simulink model "Evaporator"  (R2022b)
settings: Solver=ode45  StartTime=0.0  StopTime=30  RelTol=1e-3
undefined symbols (not defined in the file): h3, tc, tcw12
settings Model: Creator=YJT  LastModifiedBy=YJT

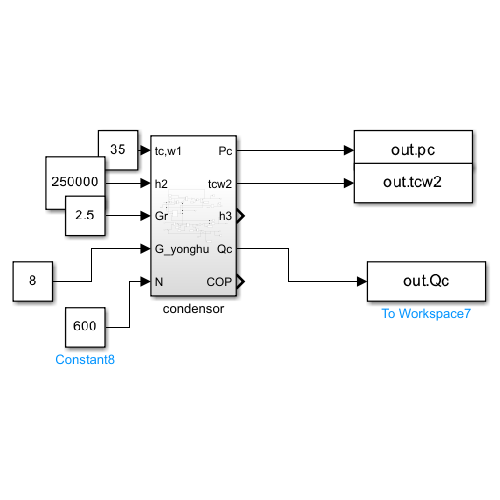
[thumbnail: Simulink's stored preview of the top-level diagram]
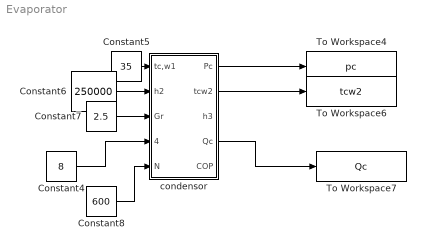
== system Evaporator ==
  Constant4 : Constant  Value=8
  Constant5 : Constant  Value=35
  Constant6 : Constant  Value=250000
  Constant7 : Constant  Value=2.5
  Constant8 : Constant  Value=600
  To Workspace4 : ToWorkspace  VariableName=pc  SaveFormat=Timeseries  SampleTime=-1
  To Workspace6 : ToWorkspace  VariableName=tcw2  SaveFormat=Timeseries  SampleTime=-1
  To Workspace7 : ToWorkspace  VariableName=Qc  SaveFormat=Timeseries  SampleTime=-1
  condensor : Subsystem
  wires:
  Constant4/1 -> condensor/4(G_yonghu)
  Constant5/1 -> condensor/1(tc,w1)
  Constant6/1 -> condensor/2(h2)
  Constant7/1 -> condensor/3(Gr)
  Constant8/1 -> condensor/5(N)
  condensor/1(Pc) -> To Workspace4/1
  condensor/4(Qc) -> To Workspace7/1
  condensor/2(tcw2) -> To Workspace6/1

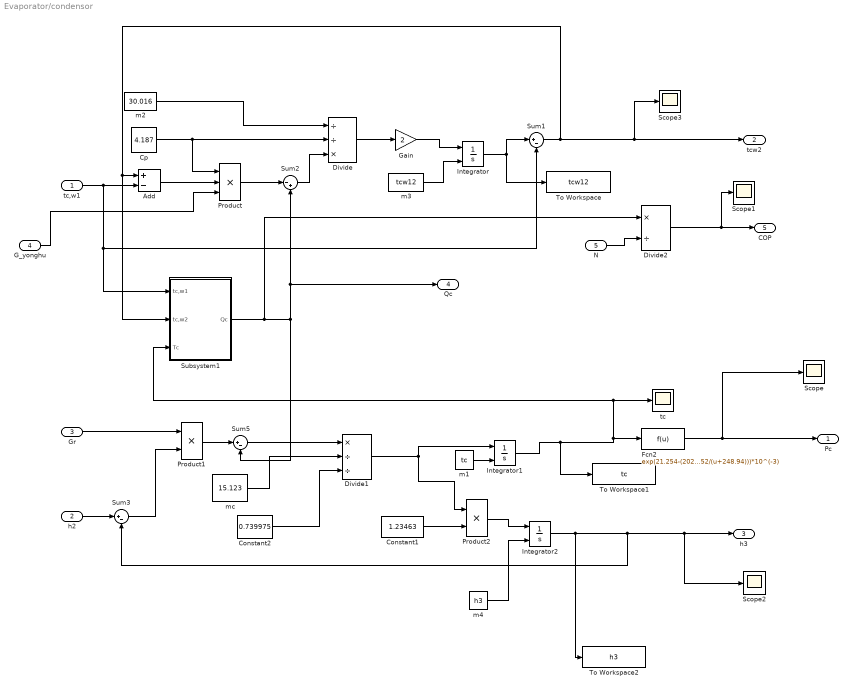
== system Evaporator/condensor ==
  tc,w1 : Inport
  h2 : Inport  Port=2
  Gr : Inport  Port=3
  G_yonghu : Inport  Port=4
  N : Inport  Port=5
  Add : Sum  Inputs=+-
  Constant1 : Constant  Value=1.23463
  Constant2 : Constant  Value=0.739975
  Cp : Constant  Value=4.187
  Divide : Product  Inputs=//*
  Divide1 : Product  Inputs=*//
  Divide2 : Product  Inputs=*/
  Fcn2 : Fcn  Expr=exp(21.254-(2025.452/(u+248.94)))*10^(-3)
  Gain : Gain  Gain=2
  Integrator : Integrator  InitialConditionSource=external
  Integrator1 : Integrator  InitialConditionSource=external
  Integrator2 : Integrator  InitialConditionSource=external
  Product : Product  Inputs=3
  Product1 : Product
  Product2 : Product
  Scope{,1..3} (4 alike) : Scope
  Subsystem1 : Subsystem
  Sum1 : Sum  Inputs=|+-
  Sum2 : Sum  Inputs=|-+
  Sum3 : Sum  Inputs=|+-
  Sum5 : Sum  Inputs=|+-
  To Workspace : ToWorkspace  VariableName=tcw12  SaveFormat=Timeseries  SampleTime=-1
  To Workspace1 : ToWorkspace  VariableName=tc  SaveFormat=Timeseries  SampleTime=-1
  To Workspace2 : ToWorkspace  VariableName=h3  SaveFormat=Timeseries  SampleTime=-1
  m1 : Constant  Value=tc
  m2 : Constant  Value=30.016
  m3 : Constant  Value=tcw12
  m4 : Constant  Value=h3
  mc : Constant  Value=15.123
  tc : Scope
  Pc : Outport
  tcw2 : Outport  Port=2
  h3 : Outport  Port=3
  Qc : Outport  Port=4
  COP : Outport  Port=5
  wires:
  Product1/1 -> Sum5/1
  Sum3/1 -> Product1/2
  Sum1/1 -> Scope3/1, tcw2/1, Subsystem1/2(tc,w2), Add/1
  Gr/1 -> Product1/1
  Integrator2/1 -> To Workspace2/1, Scope2/1, h3/1, Sum3/2
  Constant2/1 -> Divide1/3
  Gain/1 -> Integrator/1
  tc,w1/1 -> Add/2, Subsystem1/1(tc,w1), Sum1/2
  Fcn2/1 -> Scope/1, Pc/1
  Product2/1 -> Integrator2/1
  Integrator/1 -> Sum1/1, To Workspace/1
  m2/1 -> Divide/1
  Cp/1 -> Product/1, Divide/2
  Constant1/1 -> Product2/2
  G_yonghu/1 -> Product/3
  Divide1/1 -> Integrator1/1, Product2/1
  Divide/1 -> Gain/1
  h2/1 -> Sum3/1
  Product/1 -> Sum2/1
  Add/1 -> Product/2
  Sum5/1 -> Divide1/1
  Sum2/1 -> Divide/3
  mc/1 -> Divide1/2
  m1/1 -> Integrator1/2
  Integrator1/1 -> To Workspace1/1, tc/1, Subsystem1/3(Tc), Fcn2/1
  m3/1 -> Integrator/2
  m4/1 -> Integrator2/2
  Divide2/1 -> Scope1/1, COP/1
  Subsystem1/1(Qc) -> Divide2/1, Sum5/2, Qc/1, Sum2/2
  N/1 -> Divide2/2

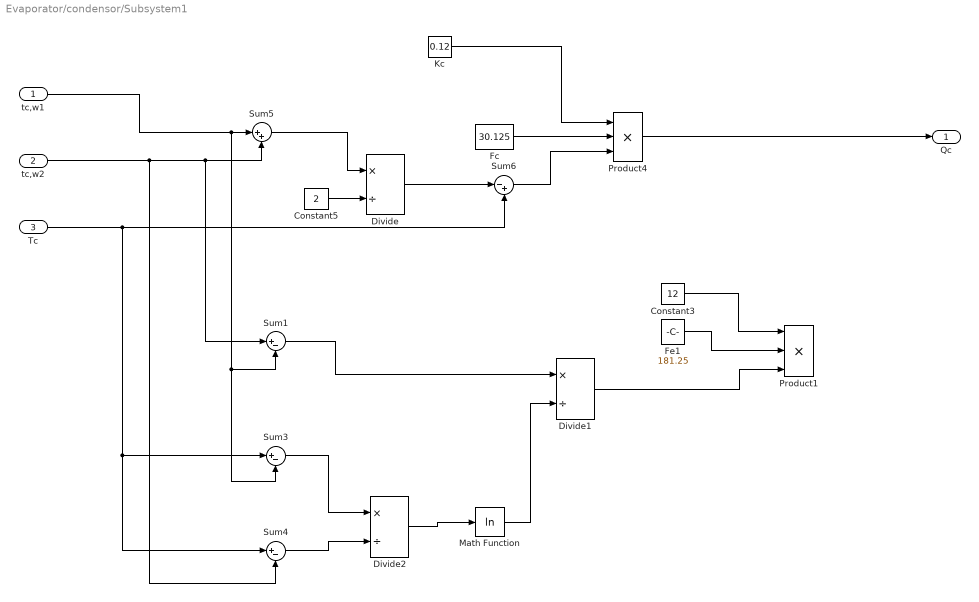
== system Evaporator/condensor/Subsystem1 ==
  tc,w1 : Inport
  tc,w2 : Inport  Port=2
  Tc : Inport  Port=3
  Constant3 : Constant  Value=12
  Constant5 : Constant  Value=2
  Divide : Product  Inputs=*/
  Divide1 : Product  Inputs=*/
  Divide2 : Product  Inputs=*/
  Fc : Constant  Value=30.125
  Fe1 : Constant  Value=181.25
  Kc : Constant  Value=0.12
  Math Function : Math  Operator=log
  Product1 : Product  Inputs=3
  Product4 : Product  Inputs=3
  Sum1 : Sum  Inputs=|+-
  Sum3 : Sum  Inputs=|+-
  Sum4 : Sum  Inputs=|+-
  Sum5 : Sum  Inputs=|++
  Sum6 : Sum  Inputs=|-+
  Qc : Outport
  wires:
  Divide/1 -> Sum6/1
  Fc/1 -> Product4/2
  Sum6/1 -> Product4/3
  Tc/1 -> Sum4/1, Sum3/1, Sum6/2
  Constant5/1 -> Divide/2
  Kc/1 -> Product4/1
  Sum5/1 -> Divide/1
  Sum3/1 -> Divide2/1
  Divide2/1 -> Math Function/1
  tc,w1/1 -> Sum3/2, Sum1/2, Sum5/1
  Sum1/1 -> Divide1/1
  Fe1/1 -> Product1/2
  Constant3/1 -> Product1/1
  Sum4/1 -> Divide2/2
  Divide1/1 -> Product1/3
  tc,w2/1 -> Sum4/2, Sum1/1, Sum5/2
  Math Function/1 -> Divide1/2
  Product4/1 -> Qc/1
